simulink model "sys_with_kalman_2016"  (R2016a)
settings: Solver=FixedStepAuto  SolverMode=SingleTasking  StartTime=0.0  StopTime=T  RelTol=1e-3
values from neighbouring files (symbols this model uses):
  A = [[-0.322, 0.052, 0.028, -1.12, 0.002], ... (first row only)    [run_task_3e.m]
  B = [0, 0, 0, 0, 10]'    [run_task_3e.m]
  C3 = [[0, 0, 0, 1, 0], ... (first row only)    [run_task_3e.m]
  D = [0, 0, 0, 0, 0]'    [run_task_3e.m]
  disturbance = 0    [run_task_3e.m]
  g = 9.81    [run_task_3e.m]
  kd = 2.153    [run_task_3e.m]
  ki = 0    [run_task_3e.m]
  kix = omega_chi^2*Vg / g    (= 0.195089817646)    [run_task_3e.m]
  kp = -1.67    [run_task_3e.m]
  kpx = 2*zeta_chi*omega_chi * Vg / g    (= 3.00138180994)    [run_task_3e.m]
  P_0 = eye(5) * 5 * deg2rad    [run_task_3e.m]
  p_noise = 0.5^2 * deg2rad^2    (= 7.61543549467e-05)    [run_task_3e.m]
  phi_noise = 2^2 * deg2rad^2    (= 0.00121846967915)    [run_task_3e.m]
  r_noise = 0.2^2 * deg2rad^2    (= 1.21846967915e-05)    [run_task_3e.m]
  samplingfrequency = 10    [run_task_3e.m]
  Tl = 0.1    [run_task_3e.m]
  Vg = 637/3.6    (= 176.944444444)    [run_task_3e.m]
  xhat_0 = [0,0,0,0,0]'    [run_task_3e.m]
libraries: simulink x3, dspsrcs4 x3
settings Model: Creator=kristkkr  LastModifiedBy=simenvg
settings DebuggingCC: SFUnexpectedBacktrackingDiag=error  SFNoUnconditionalDefaultTransitionDiag=error
settings GRTTargetCC: TargetLangStandard=C99 (ISO)  GeneratePreprocessorConditionals=Use local settings
settings ConfigComp: CovMetricSettings=dwe  CovHtmlReporting=off  CovSaveCumulativeToWorkspaceVar=off  CovSaveSingleToWorkspaceVar=off  CovExternalEMLEnable=on

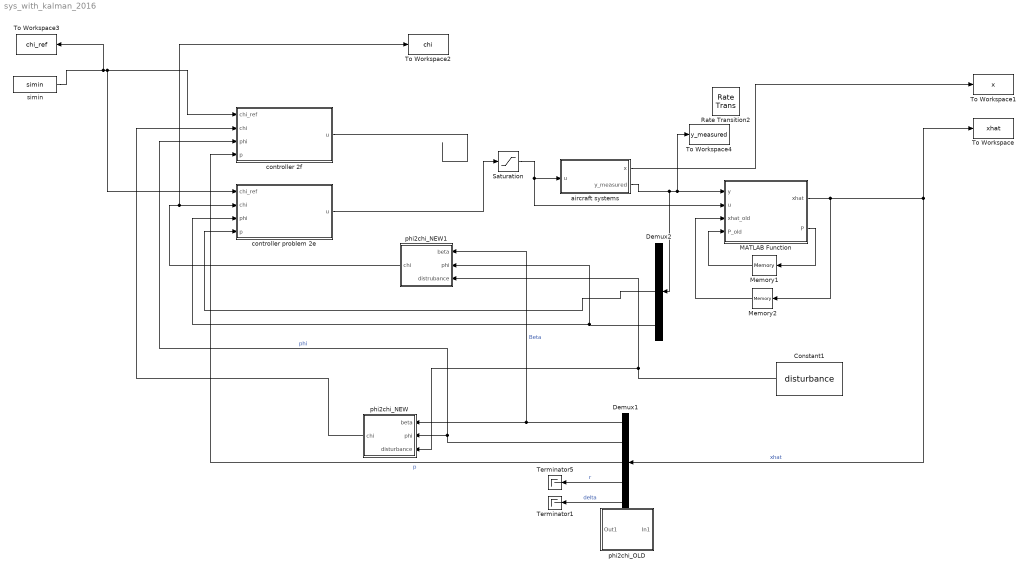
== system sys_with_kalman_2016 ==
  Constant1 : Constant  Value=disturbance
  Demux1 : Demux  Outputs=5
  Demux2 : Demux  Outputs=3
  MATLAB Function : MATLAB Function  TreatAsAtomicUnit=on
  Memory1 : Memory  X0=P_0
  Memory2 : Memory  X0=xhat_0
  Rate Transition2 : RateTransition  OutPortSampleTime=samplingfrequency
  Saturation : Saturate  UpperLimit=25*deg2rad  LowerLimit=-25*deg2rad
  Terminator1 : Terminator
  Terminator5 : Terminator
  To Workspace : ToWorkspace  VariableName=xhat  SaveFormat=Timeseries  SampleTime=-1
  To Workspace1 : ToWorkspace  VariableName=x  SaveFormat=Timeseries  SampleTime=-1
  To Workspace2 : ToWorkspace  VariableName=chi  SaveFormat=Timeseries  SampleTime=-1
  To Workspace3 : ToWorkspace  VariableName=chi_ref  SaveFormat=Timeseries  SampleTime=-1
  To Workspace4 : ToWorkspace  VariableName=y_measured  SaveFormat=Timeseries  SampleTime=-1
  aircraft systems : Subsystem
  controller 2f : Subsystem
  controller problem 2e : Subsystem
  phi2chi_NEW : Subsystem
  phi2chi_NEW1 : Subsystem
  phi2chi_OLD : Subsystem
  simin : FromWorkspace  VariableName=simin  SampleTime=0
  wires:
  MATLAB Function/1(xhat) -> Memory2/1, Demux1/1, To Workspace/1  "xhat"
  Demux1/3 -> controller 2f/4(p)  "p"
  Demux1/1 -> phi2chi_NEW/1("beta "), phi2chi_NEW1/1("beta ")  "Beta"
  Demux1/2 -> phi2chi_NEW/2(phi), controller 2f/3(phi)  "phi"
  Demux1/4 -> Terminator5/1  "r"
  Demux1/5 -> Terminator1/1  "delta"
  aircraft systems/1(x) -> To Workspace1/1
  simin/1 -> To Workspace3/1, controller problem 2e/1(chi_ref), controller 2f/1(chi_ref)
  phi2chi_NEW/1(chi) -> controller 2f/2(chi)
  aircraft systems/2(y_measured) -> Demux2/1, To Workspace4/1, MATLAB Function/1(y)
  MATLAB Function/2(P) -> Memory1/1
  Memory1/1 -> MATLAB Function/4(P_old)
  Memory2/1 -> MATLAB Function/3(xhat_old)
  Saturation/1 -> MATLAB Function/2(u), aircraft systems/1(u)
  Demux2/3 -> phi2chi_NEW1/2(phi), controller problem 2e/3(phi)
  phi2chi_NEW1/1(chi) -> To Workspace2/1, controller problem 2e/2(chi)
  Demux2/2 -> controller problem 2e/4(p)
  controller 2f/1(u) -> ?
  controller problem 2e/1(u) -> Saturation/1
  Constant1/1 -> phi2chi_NEW/3("disturbance "), phi2chi_NEW1/3(distrubance)

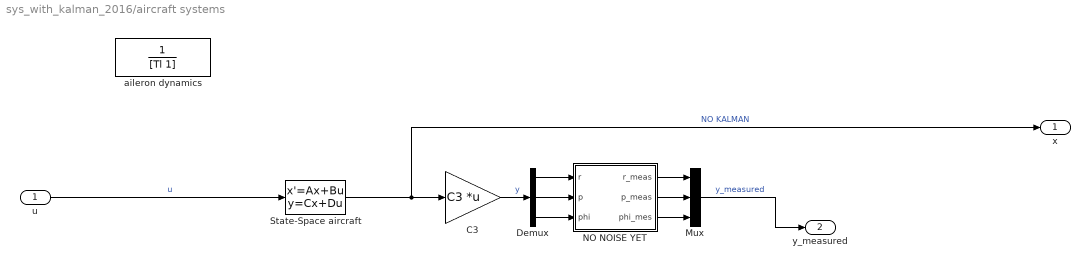
== system sys_with_kalman_2016/aircraft systems ==
  u : Inport
  C3 : Gain  Gain=C3  Multiplication=Matrix(K*u) (u vector)
  Demux : Demux  Outputs=3
  Mux : Mux  Inputs=3
  NO NOISE YET : Subsystem
  State-Space aircraft : StateSpace  A=A  B=B  C=eye(5)  D=D  X0=0
  aileron dynamics : TransferFcn  Denominator=[Tl 1]
  x : Outport
  y_measured : Outport  Port=2
  wires:
  u/1 -> State-Space aircraft/1  "u"
  Mux/1 -> y_measured/1  "y_measured"
  NO NOISE YET/2(p_meas) -> Mux/2
  NO NOISE YET/3(phi_mes) -> Mux/3
  C3/1 -> Demux/1  "y"
  State-Space aircraft/1 -> x/1, C3/1  "NO KALMAN"
  NO NOISE YET/1(r_meas) -> Mux/1
  Demux/1 -> NO NOISE YET/1(r)
  Demux/2 -> NO NOISE YET/2(p)
  Demux/3 -> NO NOISE YET/3(phi)
  ? -> ?

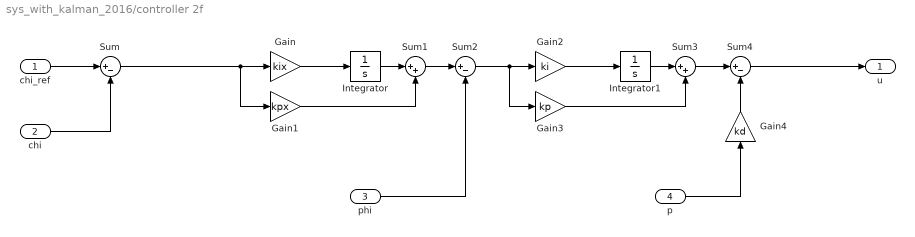
== system sys_with_kalman_2016/controller 2f ==
  chi_ref : Inport
  chi : Inport  Port=2
  phi : Inport  Port=3
  p : Inport  Port=4
  Gain : Gain  Gain=kix
  Gain1 : Gain  Gain=kpx
  Gain2 : Gain  Gain=ki
  Gain3 : Gain  Gain=kp
  Gain4 : Gain  Gain=kd
  Integrator : Integrator
  Integrator1 : Integrator
  Sum : Sum  Inputs=|+-
  Sum1 : Sum  Inputs=|++
  Sum2 : Sum  Inputs=|+-
  Sum3 : Sum  Inputs=|++
  Sum4 : Sum  Inputs=|+-
  u : Outport
  wires:
  Sum1/1 -> Sum2/1
  Sum2/1 -> Gain3/1, Gain2/1
  Sum3/1 -> Sum4/1
  Sum/1 -> Gain1/1, Gain/1
  chi_ref/1 -> Sum/1
  Integrator/1 -> Sum1/1
  Gain4/1 -> Sum4/2
  Gain/1 -> Integrator/1
  Gain2/1 -> Integrator1/1
  Integrator1/1 -> Sum3/1
  Gain1/1 -> Sum1/2
  Gain3/1 -> Sum3/2
  chi/1 -> Sum/2
  p/1 -> Gain4/1
  phi/1 -> Sum2/2
  Sum4/1 -> u/1

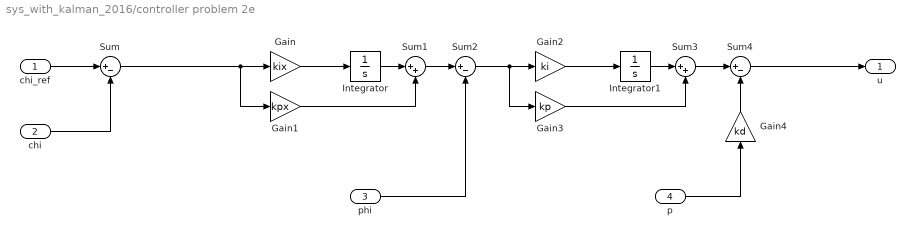
== system sys_with_kalman_2016/controller problem 2e ==
  chi_ref : Inport
  chi : Inport  Port=2
  phi : Inport  Port=3
  p : Inport  Port=4
  Gain : Gain  Gain=kix
  Gain1 : Gain  Gain=kpx
  Gain2 : Gain  Gain=ki
  Gain3 : Gain  Gain=kp
  Gain4 : Gain  Gain=kd
  Integrator : Integrator
  Integrator1 : Integrator
  Sum : Sum  Inputs=|+-
  Sum1 : Sum  Inputs=|++
  Sum2 : Sum  Inputs=|+-
  Sum3 : Sum  Inputs=|++
  Sum4 : Sum  Inputs=|+-
  u : Outport
  wires:
  Sum1/1 -> Sum2/1
  Sum2/1 -> Gain3/1, Gain2/1
  Sum3/1 -> Sum4/1
  Sum/1 -> Gain1/1, Gain/1
  chi_ref/1 -> Sum/1
  Integrator/1 -> Sum1/1
  Gain4/1 -> Sum4/2
  Gain/1 -> Integrator/1
  Gain2/1 -> Integrator1/1
  Integrator1/1 -> Sum3/1
  Gain1/1 -> Sum1/2
  Gain3/1 -> Sum3/2
  chi/1 -> Sum/2
  p/1 -> Gain4/1
  phi/1 -> Sum2/2
  Sum4/1 -> u/1

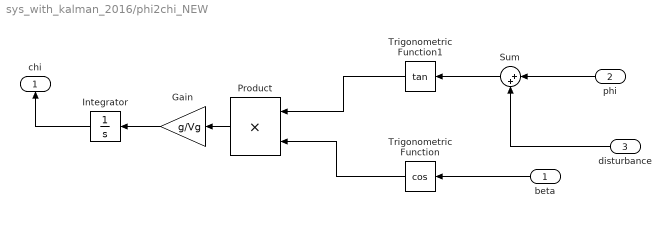
== system sys_with_kalman_2016/phi2chi_NEW ==
  "beta " : Inport
  phi : Inport  Port=2
  "disturbance " : Inport  Port=3
  Gain : Gain  Gain=g/Vg
  Integrator : Integrator
  Product : Product
  Sum : Sum  Inputs=|++
  Trigonometric Function : Trigonometry  Operator=cos
  Trigonometric Function1 : Trigonometry  Operator=tan
  chi : Outport
  wires:
  Integrator/1 -> chi/1
  Product/1 -> Gain/1
  "beta "/1 -> Trigonometric Function/1
  Gain/1 -> Integrator/1
  Trigonometric Function1/1 -> Product/1
  Trigonometric Function/1 -> Product/2
  Sum/1 -> Trigonometric Function1/1
  phi/1 -> Sum/1
  "disturbance "/1 -> Sum/2

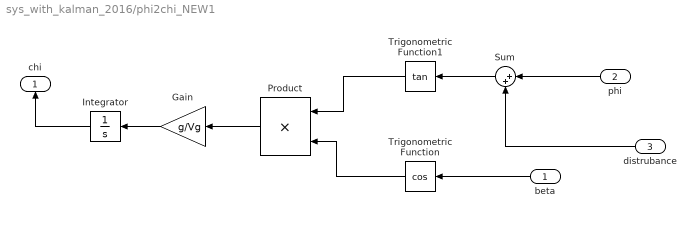
== system sys_with_kalman_2016/phi2chi_NEW1 ==
  "beta " : Inport
  phi : Inport  Port=2
  distrubance : Inport  Port=3
  Gain : Gain  Gain=g/Vg
  Integrator : Integrator
  Product : Product
  Sum : Sum  Inputs=|++
  Trigonometric Function : Trigonometry  Operator=cos
  Trigonometric Function1 : Trigonometry  Operator=tan
  chi : Outport
  wires:
  Integrator/1 -> chi/1
  phi/1 -> Sum/1
  Product/1 -> Gain/1
  "beta "/1 -> Trigonometric Function/1
  Gain/1 -> Integrator/1
  Trigonometric Function1/1 -> Product/1
  Trigonometric Function/1 -> Product/2
  distrubance/1 -> Sum/2
  Sum/1 -> Trigonometric Function1/1

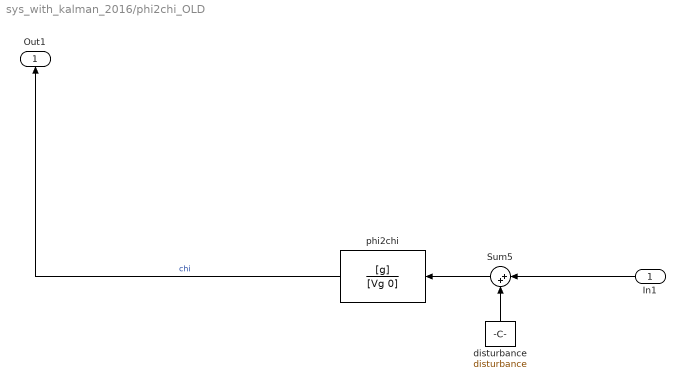
== system sys_with_kalman_2016/phi2chi_OLD ==
  In1 : Inport
  Sum5 : Sum  Inputs=|++
  disturbance : Constant  Value=disturbance
  phi2chi : TransferFcn  Numerator=[g]  Denominator=[Vg 0]
  Out1 : Outport
  wires:
  In1/1 -> Sum5/1
  phi2chi/1 -> Out1/1  "chi"
  disturbance/1 -> Sum5/2
  Sum5/1 -> phi2chi/1

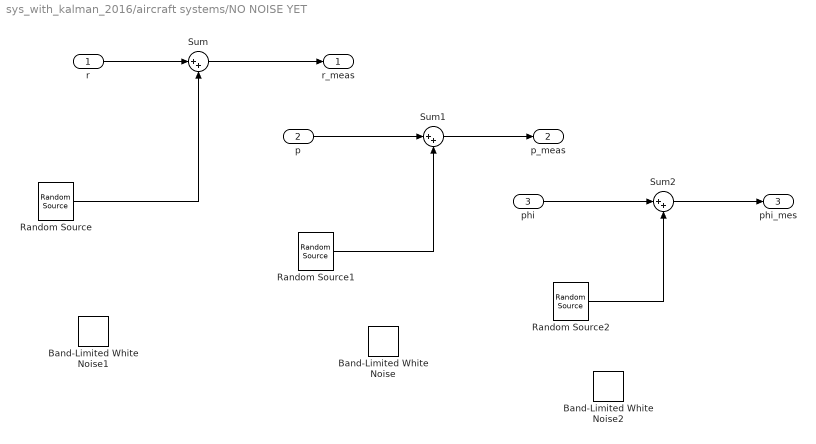
== system sys_with_kalman_2016/aircraft systems/NO NOISE YET ==
  r : Inport
  p : Inport  Port=2
  phi : Inport  Port=3
  Band-Limited White Noise : simulink/Sources/Band-Limited White Noise  Cov=[p_noise]  Ts=0.1  seed=[23341]
  Band-Limited White Noise1 : simulink/Sources/Band-Limited White Noise  Cov=[r_noise]  Ts=0.1  seed=[23341]
  Band-Limited White Noise2 : simulink/Sources/Band-Limited White Noise  Cov=[phi_noise]  Ts=0.1  seed=[23341]
  Random Source : dspsrcs4/Random Source  SrcType=Gaussian  NormMethod=Ziggurat  CltLength=12  MinVal=0  MaxVal=1  MeanVal=0  VarVal=r_noise  RepMode=Not repeatable  rawSeed=1  IsInherit=off  SampMode=Discrete  SampTime=1/samplingfrequency  SampFrame=1  DataType=Double  OutComplex=Real  OutputFrames=off
  Random Source1 : dspsrcs4/Random Source  SrcType=Gaussian  NormMethod=Ziggurat  CltLength=12  MinVal=0  MaxVal=1  MeanVal=0  VarVal=p_noise  RepMode=Not repeatable  rawSeed=1  IsInherit=off  SampMode=Discrete  SampTime=1/samplingfrequency  SampFrame=1  DataType=Double  OutComplex=Real  OutputFrames=off
  Random Source2 : dspsrcs4/Random Source  SrcType=Gaussian  NormMethod=Ziggurat  CltLength=12  MinVal=0  MaxVal=1  MeanVal=0  VarVal=phi_noise  RepMode=Not repeatable  rawSeed=1  IsInherit=off  SampMode=Discrete  SampTime=1/samplingfrequency  SampFrame=1  DataType=Double  OutComplex=Real  OutputFrames=off
  Sum : Sum  Inputs=|++
  Sum1 : Sum  Inputs=|++
  Sum2 : Sum  Inputs=|++
  r_meas : Outport
  p_meas : Outport  Port=2
  phi_mes : Outport  Port=3
  wires:
  p/1 -> Sum1/1
  r/1 -> Sum/1
  Sum/1 -> r_meas/1
  Sum1/1 -> p_meas/1
  Sum2/1 -> phi_mes/1
  phi/1 -> Sum2/1
  Random Source2/1 -> Sum2/2
  Random Source1/1 -> Sum1/2
  Random Source/1 -> Sum/2

== matlab function sys_with_kalman_2016/MATLAB Function ==
  data: y input; u input; xhat_old input; P_old input; xhat output; P output
function [xhat, P]  = kalman_filter(y,u, xhat_old, P_old)

vars = load('vars.mat');
%vars2 = load('vars2.mat');


x_predicted = vars.A_d*xhat_old + vars.B_d*u;
P_predicted = vars.A_d*P_old*vars.A_d' + vars.Q;

K_gain = P_predicted*vars.H'*inv(vars.H*P_predicted*vars.H' + vars.R);
xhat = x_predicted + K_gain*(y - vars.H*x_predicted);
P = (eye(5) - K_gain*vars.H)*P_predicted;
